simulink model "VectorCalc"  (R2021a)
settings: Solver=FixedStepDiscrete  StartTime=0.0  StopTime=10.0  RelTol=1e-3  EnableMultiTasking=on
settings Model: Creator=Mina  LastModifiedBy=Mina
settings DataIOCC: ReturnWorkspaceOutputs=off
settings OptimizationCC: DefaultParameterBehavior=Inlined  InlineInvariantSignals=on  EnableMemcpy=off  LifeSpan=1  EfficientTunableParamExpr=on
settings DebuggingCC: UnderspecifiedInitializationDetection=Classic  MergeDetectMultiDrivingBlocksExec=none  SFMachineParentedDataDiag=warning  ArithmeticOperatorsInVariantConditions=warning
settings ModelReferenceCC: PropagateSignalLabelsOutOfModel=off
settings SFSimCC: MATLABDynamicMemAlloc=off  CustomCodeUndefinedFunction=UseInterfaceOnly
settings RTWCC: SystemTargetFile=ert.tlc  GenCodeOnly=on  TemplateMakefile=ert_default_tmf  GenerateReport=on  IncludeHyperlinkInReport=on  LaunchReport=on  GenerateTraceInfo=on  GenerateTraceReport=on  GenerateTraceReportSl=on  GenerateTraceReportSf=on  GenerateTraceReportEml=on
settings CodeAppCC: ForceParamTrailComments=on  IgnoreCustomStorageClasses=off  OperatorAnnotations=on  SimulinkDataObjDesc=on  SFDataObjDesc=on  MATLABFcnDesc=on  InsertBlockDesc=on  StateflowObjectComments=on  MATLABSourceComments=on
settings ERTTargetCC: MultiwordLength=2048  GenerateSampleERTMain=on  InlinedParameterPlacement=NonHierarchical  ERTCustomFileTemplate=example_file_process.tlc

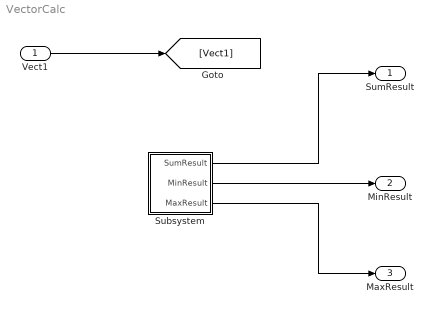
== system VectorCalc ==
  Vect1 : Inport  OutDataTypeStr=uint8  PortDimensions=3
  Subsystem : Subsystem
  SumResult : Outport
  MinResult : Outport  Port=2
  MaxResult : Outport  Port=3
  wires:
  Vect1/1 -> [Vect1]
  Subsystem/1(SumResult) -> SumResult/1
  Subsystem/2(MinResult) -> MinResult/1
  Subsystem/3(MaxResult) -> MaxResult/1

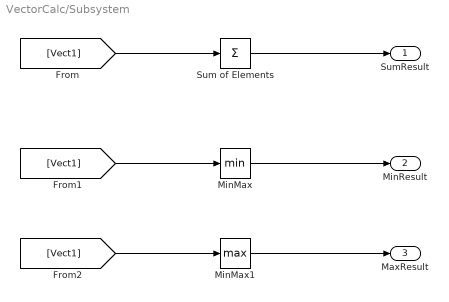
== system VectorCalc/Subsystem ==
  MinMax : MinMax
  MinMax1 : MinMax  Function=max
  Sum of Elements : Sum  Inputs=+
  SumResult : Outport
  MinResult : Outport  Port=2
  MaxResult : Outport  Port=3
  wires:
  [Vect1] -> MinMax1/1
  [Vect1] -> Sum of Elements/1
  Sum of Elements/1 -> SumResult/1
  MinMax/1 -> MinResult/1
  MinMax1/1 -> MaxResult/1
  [Vect1] -> MinMax/1
